simulink model "Sim_OSQP_PC"  (R2025b)
settings: Solver=ode45  StartTime=0.0  StopTime=0.7  FixedStep=Ts/2  RelTol=1e-3
values from neighbouring files (symbols this model uses):
  Ad = evalin('base','Ad')    [PC_OSQP.m]    (also in PC_OSQP_WHAT.m)
  Bd = evalin('base','Bd')    [PC_OSQP.m]    (also in PC_OSQP_WHAT.m)
  Cf = Cf_values(k)    [Init_OSQP_PC.m]    (also in PC_PIControl.m = 1.2e-05)
  Lf = Lf_values(k)    [Init_OSQP_PC.m]    (also in PC_PIControl.m = 0.005)
  Lg = Lg_values(k)    [Init_OSQP_PC.m]    (also in PC_PIControl.m = 0.0033)
  Rf = 0.035    [Init_OSQP_PC.m]    (also in PC_PIControl.m)
  Rg = Rg_values(k)    [Init_OSQP_PC.m]    (also in PC_PIControl.m = 0.84)
  Ts = 1/fs    (= 0.0002)    [Init_OSQP_PC.m]    (also in PC_PIControl.m)
  Vb = Vdc*(sqrt(3)/3)/1.15    [Init_OSQP_PC.m]    (also in PC_PIControl.m)
  Vdc = 300    [Init_OSQP_PC.m]    (also in PC_PIControl.m)
  wb = 2*pi*f    (= 314.159265359)    [Init_OSQP_PC.m]    (also in PC_PIControl.m)
undefined symbols (not defined in the file or in its folder): Bpd, Cd, plecs
libraries: dspsigops x2
settings Model: Creator=ASUS-PC  LastModifiedBy=dfigueroa
settings SolverCC: AllowMultiTaskInputOutput=on  PositivePriorityOrder=on
settings DebuggingCC: IntegerOverflowMsg=error  ParameterPrecisionLossMsg=error  UnderSpecifiedDimensionMsg=warning
settings RTWCC: GPUComputeCapability=3.5

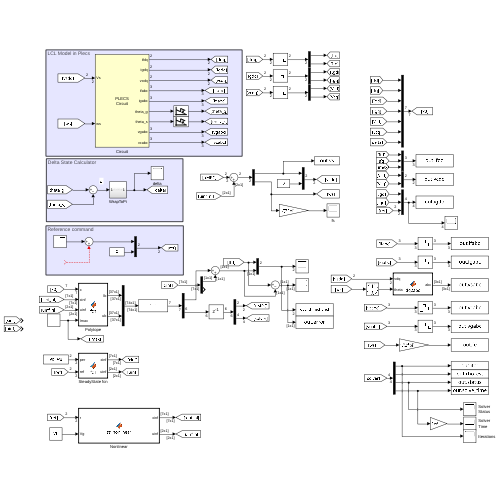
[thumbnail: Simulink's stored preview of the top-level diagram]
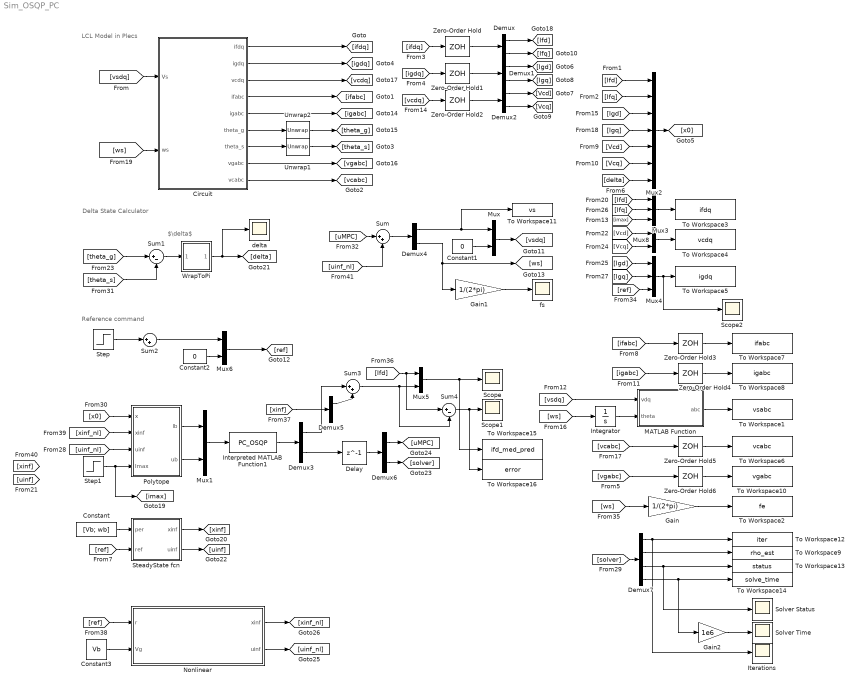
== system Sim_OSQP_PC ==
  note: LCL Model in Plecs
  note: Reference command
  note: $\delta$
  note: Delta State Calculator
  Circuit : Subsystem  LoadFcn=plecs('sl', 200);  InitFcn=plecs('sl', 214);  StartFcn=plecs('sl', 208);  StopFcn=plecs('sl', 209);  mask(PlecsCircuit){PLECSData=<binary blob, 7204 chars, not shown>}
      mask prompts: PLECSData "PLECS Data (Do not delete or modify!)"
      mask init:
      | % PLACE CUSTOM INITIALIZATIONS ABOVE
      | % DO NOT REMOVE
      | plecs('sl', 215);
      | % DO NOT REMOVE
      settings: CopyFcn=plecs('sl', 203);  DeleteFcn=plecs('sl', 205);  UndoDeleteFcn=plecs('sl', 206);  PreSaveFcn=plecs('sl', 211);  PostSaveFcn=plecs('sl', 201);  NameChangeFcn=plecs('sl', 210);  DestroyFcn=plecs('sl', 207);  PreCopyFcn=plecs('sl', 216);  OpenFcn=plecs('sl', 202);  ErrorFcn=plerrorfcn
      mask Help: eval('plecs(''help'', ''qthelp:///creatingacircuit.html'')')
      mask Display: disp('PLECS\nCircuit')
  Constant : Constant  Value=[Vb; wb]  SampleTime=Ts
  Constant1 : Constant  Value=0  SampleTime=Ts
  Constant2 : Constant  Value=0  SampleTime=Ts
  Constant3 : Constant  Value=Vb
  Delay : Delay  DelayLength=1  InitialCondition=0  SampleTime=Ts
  Demux{,1..2,4} (4 alike) : Demux  Outputs=2
  Demux3 : Demux  Outputs=[1;6]
  Demux5 : Demux  Outputs=[1;6]
  Demux6 : Demux  Outputs=[2;4]
  Demux7 : Demux
  Gain : Gain  Gain=1/(2*pi)
  Gain1 : Gain  Gain=1/(2*pi)
  Gain2 : Gain  Gain=1e6
  Integrator : Integrator  WrapState=on
  Interpreted MATLAB Function1 : MATLABFcn  StartFcn=clear PC_OSQP  MATLABFcn=PC_OSQP  OutputDimensions=7
  Iterations : Scope
      settings: Title=Iterations  ActiveDisplayYMinimum=-3.75  ActiveDisplayYMaximum=33.75  YLabel=Iterations Number [-]
  MATLAB Function : MATLAB Function  TreatAsAtomicUnit=on
  Mux{,1,5..6,8} (5 alike) : Mux  Inputs=2
  Mux2 : Mux  Inputs=7
  Mux3 : Mux  Inputs=3
  Mux4 : Mux  Inputs=3
  Nonlinear : MATLAB Function  TreatAsAtomicUnit=on
  Polytope : MATLAB Function  TreatAsAtomicUnit=on
  Scope : Scope
      settings: ActiveDisplayYMinimum=-4.5545615046409651  ActiveDisplayYMaximum=8.000947565725788
  Scope1 : Scope
      settings: ActiveDisplayYMinimum=-0.52018876993310137  ActiveDisplayYMaximum=1.1247691139620895  DataLoggingVariableName=ScopeData6
  Scope2 : Scope
      settings: ActiveDisplayYMinimum=2.349689265196981  ActiveDisplayYMaximum=6.2165319723258836  DataLoggingVariableName=ScopeData7
  Solver Status : Scope
      settings: ActiveDisplayYMinimum=-2.5  ActiveDisplayYMaximum=2.5  DataLoggingVariableName=ScopeData2
  Solver Time : Scope
      settings: Title=Solver Timer  ActiveDisplayYMinimum=-35.6125  ActiveDisplayYMaximum=320.5125  YLabel=Solver Time [\mu s]  DataLoggingVariableName=ScopeData3
  SteadyState fcn : MATLAB Function  TreatAsAtomicUnit=on
  Step : Step  Time=0.2  Before=3  After=5.5  SampleTime=Ts
  Step1 : Step  Time=0.4  Before=7  After=4  SampleTime=Ts
  Sum : Sum  Inputs=|++
  Sum1 : Sum  Inputs=|+-
  Sum2 : Sum  Inputs=|++
  Sum3 : Sum  Inputs=|++
  Sum4 : Sum  Inputs=|+-
  To Workspace1 : ToWorkspace  VariableName=vsabc  SaveFormat=Structure With Time  SampleTime=Ts
  To Workspace10 : ToWorkspace  VariableName=vgabc  SaveFormat=Structure With Time  SampleTime=Ts
  To Workspace11 : ToWorkspace  VariableName=vs  SaveFormat=Structure With Time  SampleTime=Ts
  To Workspace12 : ToWorkspace  VariableName=iter  SaveFormat=Structure With Time  SampleTime=Ts
  To Workspace13 : ToWorkspace  VariableName=status  SaveFormat=Structure With Time  SampleTime=Ts
  To Workspace14 : ToWorkspace  VariableName=solve_time  SaveFormat=Structure With Time  SampleTime=Ts
  To Workspace15 : ToWorkspace  VariableName=ifd_med_pred  SaveFormat=Structure With Time  SampleTime=Ts
  To Workspace16 : ToWorkspace  VariableName=error  SaveFormat=Structure With Time  SampleTime=Ts
  To Workspace2 : ToWorkspace  VariableName=fe  SaveFormat=Structure With Time  SampleTime=Ts
  To Workspace3 : ToWorkspace  VariableName=ifdq  SaveFormat=Structure With Time  SampleTime=Ts
  To Workspace4 : ToWorkspace  VariableName=vcdq  SaveFormat=Structure With Time  SampleTime=Ts
  To Workspace5 : ToWorkspace  VariableName=igdq  SaveFormat=Structure With Time  SampleTime=Ts
  To Workspace6 : ToWorkspace  VariableName=vcabc  SaveFormat=Structure With Time  SampleTime=Ts
  To Workspace7 : ToWorkspace  VariableName=ifabc  SaveFormat=Structure With Time  SampleTime=Ts
  To Workspace8 : ToWorkspace  VariableName=igabc  SaveFormat=Structure With Time  SampleTime=Ts
  To Workspace9 : ToWorkspace  VariableName=rho_est  SaveFormat=Structure With Time  SampleTime=Ts
  Unwrap1 : dspsigops/Unwrap  tol=pi  InputProcessing=Columns as channels (frame based)  running=off
  Unwrap2 : dspsigops/Unwrap  tol=pi  InputProcessing=Columns as channels (frame based)  running=off
  WrapToPi : Subsystem
  Zero-Order Hold{,1..6} (7 alike) : ZeroOrderHold  SampleTime=Ts
  delta : Scope
      settings: ActiveDisplayYMinimum=-1.786361940760036  ActiveDisplayYMaximum=0.36929419889135839  DataLoggingVariableName=ScopeData4
  fs : Scope
      settings: ActiveDisplayYMinimum=43.68062  ActiveDisplayYMaximum=55.78728  DataLoggingVariableName=ScopeData5
  wires:
  [Ifd] -> Mux2/1
  Circuit/8(vgabc) -> [vgabc]
  Circuit/2(igdq) -> [igdq]
  [vsdq] -> Circuit/1(Vs)
  [Vcd] -> Mux2/5
  Circuit/1(ifdq) -> [ifdq]
  Unwrap2/1 -> [theta_g]
  Circuit/5(igabc) -> [igabc]
  Circuit/3(vcdq) -> [vcdq]
  Mux2/1 -> [x0]
  [Ifq] -> Mux2/2
  [ws] -> Circuit/2(ws)
  [Vcq] -> Mux2/6
  [delta] -> Mux2/7
  Unwrap1/1 -> [theta_s]
  Circuit/4(ifabc) -> [ifabc]
  [Igq] -> Mux2/4
  [Igd] -> Mux2/3
  Constant/1 -> SteadyState fcn/1(per)
  [ref] -> SteadyState fcn/2(ref)
  [x0] -> Polytope/1(x)
  Polytope/1(lb) -> Mux1/1
  Polytope/2(ub) -> Mux1/2
  Mux1/1 -> Interpreted MATLAB Function1/1
  Circuit/9(vcabc) -> [vcabc]
  Circuit/6(theta_g) -> Unwrap2/1
  Circuit/7(theta_s) -> Unwrap1/1
  Step1/1 -> [imax], Polytope/4(Imax)
  [theta_s] -> Sum1/2
  Demux7/3 -> Solver Status/1, To Workspace13/1
  Gain2/1 -> Solver Time/1
  Sum/1 -> Demux4/1
  Constant1/1 -> Mux/2
  Gain1/1 -> fs/1
  Sum1/1 -> WrapToPi/1(In1)
  Demux7/4 -> Gain2/1, To Workspace14/1
  Demux4/2 -> Gain1/1, [ws]
  Constant2/1 -> Mux6/2
  Demux7/2 -> To Workspace9/1
  Mux/1 -> [vsdq]
  [theta_g] -> Sum1/1
  Demux7/1 -> Iterations/1, To Workspace12/1
  Mux6/1 -> [ref]
  WrapToPi/1(Out1) -> [delta], delta/1
  Delay/1 -> Demux6/1
  Demux4/1 -> To Workspace11/1, Mux/1
  Zero-Order Hold2/1 -> Demux2/1
  Demux1/2 -> [Igq]
  [vcdq] -> Zero-Order Hold2/1
  Zero-Order Hold1/1 -> Demux1/1
  Demux/1 -> [Ifd]
  Demux2/2 -> [Vcq]
  [ifdq] -> Zero-Order Hold/1
  Demux1/1 -> [Igd]
  Zero-Order Hold/1 -> Demux/1
  Demux2/1 -> [Vcd]
  [igdq] -> Zero-Order Hold1/1
  Demux/2 -> [Ifq]
  [Igq] -> Mux4/2
  [Vcd] -> Mux8/1
  Zero-Order Hold4/1 -> To Workspace8/1
  Gain/1 -> To Workspace2/1
  Zero-Order Hold3/1 -> To Workspace7/1
  Integrator/1 -> MATLAB Function/2(theta)
  [Vcq] -> Mux8/2
  Mux4/1 -> Scope2/1, To Workspace5/1
  [ifabc] -> Zero-Order Hold3/1
  [igabc] -> Zero-Order Hold4/1
  [Ifd] -> Mux3/1
  [ref] -> Mux4/3
  [vgabc] -> Zero-Order Hold6/1
  [Igd] -> Mux4/1
  MATLAB Function/1(abc) -> To Workspace1/1
  [vcabc] -> Zero-Order Hold5/1
  [Ifq] -> Mux3/2
  Zero-Order Hold6/1 -> To Workspace10/1
  [imax] -> Mux3/3
  Zero-Order Hold5/1 -> To Workspace6/1
  Mux3/1 -> To Workspace3/1
  Mux8/1 -> To Workspace4/1
  [ws] -> Integrator/1
  Step/1 -> Sum2/1
  Sum2/1 -> Mux6/1
  ? -> Sum2/2
  [vsdq] -> MATLAB Function/1(vdq)
  SteadyState fcn/1(xinf) -> [xinf]
  SteadyState fcn/2(uinf) -> [uinf]
  [xinf_nl] -> Polytope/2(xinf)
  [uinf_nl] -> Polytope/3(uinf)
  Demux6/2 -> [solver]
  [solver] -> Demux7/1
  Demux6/1 -> [uMPC]
  [uMPC] -> Sum/1
  [uinf_nl] -> Sum/2
  [ws] -> Gain/1
  Interpreted MATLAB Function1/1 -> Demux3/1
  Demux3/2 -> Delay/1
  Demux3/1 -> Sum3/1
  Mux5/1 -> To Workspace15/1, Scope/1
  Sum3/1 -> Sum4/2, Mux5/2
  [xinf] -> Demux5/1
  Demux5/1 -> Sum3/2
  Sum4/1 -> To Workspace16/1, Scope1/1
  [Ifd] -> Sum4/1, Mux5/1
  [ref] -> Nonlinear/1(r)
  Constant3/1 -> Nonlinear/2(Vg)
  Nonlinear/2(uinf) -> [uinf_nl]
  Nonlinear/1(xinf) -> [xinf_nl]

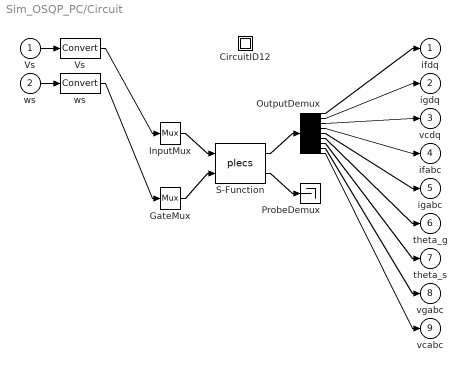
== system Sim_OSQP_PC/Circuit ==
  Vs : Inport  PortDimensions=2
  ws : Inport  Port=2  PortDimensions=1
  " CircuitID12 " : Subsystem
  " GateMux " : Mux  Inputs=[ 1 ]
  " InputMux " : Mux  Inputs=[ 2 ]
  " OutputDemux " : Demux  Outputs=[ 2 2 2 3 3 1 1 3 3 ]
  " ProbeDemux " : Terminator
  " S-Function " : S-Function  FunctionName=plecs  SFunctionDeploymentMode=off  EnableBusSupport=off
  " Vs " : DataTypeConversion
  " ws " : DataTypeConversion
  ifdq : Outport  PortDimensions=2
  igdq : Outport  Port=2  PortDimensions=2
  vcdq : Outport  Port=3  PortDimensions=2
  ifabc : Outport  Port=4  PortDimensions=3
  igabc : Outport  Port=5  PortDimensions=3
  theta_g : Outport  Port=6  PortDimensions=1
  theta_s : Outport  Port=7  PortDimensions=1
  vgabc : Outport  Port=8  PortDimensions=3
  vcabc : Outport  Port=9  PortDimensions=3
  wires:
  " InputMux "/1 -> " S-Function "/1
  " GateMux "/1 -> " S-Function "/2
  " S-Function "/1 -> " OutputDemux "/1
  " S-Function "/2 -> " ProbeDemux "/1
  Vs/1 -> " Vs "/1
  " Vs "/1 -> " InputMux "/1
  ws/1 -> " ws "/1
  " ws "/1 -> " GateMux "/1
  " OutputDemux "/1 -> ifdq/1
  " OutputDemux "/2 -> igdq/1
  " OutputDemux "/3 -> vcdq/1
  " OutputDemux "/4 -> ifabc/1
  " OutputDemux "/5 -> igabc/1
  " OutputDemux "/6 -> theta_g/1
  " OutputDemux "/7 -> theta_s/1
  " OutputDemux "/8 -> vgabc/1
  " OutputDemux "/9 -> vcabc/1

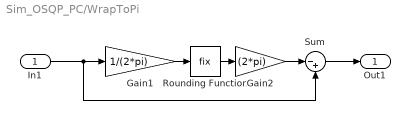
== system Sim_OSQP_PC/WrapToPi ==
  In1 : Inport
  Gain1 : Gain  Gain=1/(2*pi)
  Gain2 : Gain  Gain=(2*pi)
  Rounding Function : Rounding  Operator=fix
  Sum : Sum  Inputs=|-+
  Out1 : Outport
  wires:
  Gain2/1 -> Sum/1
  Gain1/1 -> Rounding Function/1
  Rounding Function/1 -> Gain2/1
  In1/1 -> Sum/2, Gain1/1
  Sum/1 -> Out1/1

== system Sim_OSQP_PC/Circuit/ CircuitID12  ==

== matlab function Sim_OSQP_PC/MATLAB Function ==
  data: vdq input; abc output; theta input
function abc = dq2abc(vdq,theta)
    T = [sin(theta)        -sin(theta)        ;
         cos(theta-2*pi/3) -sin(theta-2*pi/3) ;
         cos(theta+2*pi/3) -sin(theta+2*pi/3)];
    abc = T*vdq;

== matlab function Sim_OSQP_PC/Polytope ==
  data: x input; xinf input; lb output; ub output; uinf input; Imax input; Bd parameter; Vdc parameter
function [lb, ub] = fcn(x, xinf, uinf, Imax, Bd, Vdc)
    [nx,~] = size(Bd); N = 2;

    Mi = [1 0 0 0 0 0 0;
          0 1 0 0 0 0 0];

    a1 = tan(deg2rad(15)); a2 = tan(deg2rad(45)); a3 = tan(deg2rad(75));

    r1 = 1; r2 = 1.366; r3 = 3.7321;
    
    Hi = [a1  1 ;
          a2  1 ;
          a3  1 ;
          a3 -1 ;
          a2 -1 ;
          a1 -1];
 
    xmax = Imax*[r1;
                 r2;
                 r3;
                 r3;
                 r2;
                 r1];
    xmin = -xmax;

    Hv = [1 0 ;
          0 1];
    wmax = 2*pi*70;

    hv = [0.95*(sqrt(3)/3)*Vdc ;
                          wmax];
    
    umax = hv;

    umin = -umax;
    umin(2) = 0 ;

    leq = [-(x - xinf)     ;
            zeros(N*nx, 1)];
    ueq = leq;

    x_uineq = [kron(ones(N,1), xmax - Hi*Mi*xinf)];
    u_uineq = [kron(ones(N,1), umax - Hv*uinf)]   ;
    x_lineq = [kron(ones(N,1), xmin - Hi*Mi*xinf)];
    u_lineq = [kron(ones(N,1), umin - Hv*uinf)]   ;

    lb = [leq     ;
          x_lineq ;
          u_lineq];
    ub = [ueq     ;
          x_uineq ;
          u_uineq];
end

== matlab function Sim_OSQP_PC/SteadyState fcn ==
  data: per input; xinf output; uinf output; ref input; Ad parameter; Cd parameter; Bd parameter; Bpd parameter
function [xinf, uinf] = fcn(per, ref, Ad, Cd, Bd, Bpd)
    H_k = [0 0 1 0 0 0 0;
           0 0 0 1 0 0 0];
    Asolve = [eye(length(Ad)) - Ad   -Bd; 
                    H_k*Cd          zeros(size(Bd,2))];
    Csolve = [ [Bd Bpd]*[0;0;per];
                       ref];
    infty  = linsolve(Asolve,Csolve);
    xinf = infty(1:size(Ad,1));
    uinf = infty(size(Ad,1) + 1:end);
end

== matlab function Sim_OSQP_PC/Nonlinear ==
  data: r input; xinf output; uinf output; Vg input; wb parameter; Lf parameter; Rf parameter; Lg parameter; Rg parameter; Cf parameter
function [xinf, uinf] = ss_nonlinear(r, Vg, wb,Lf,Rf, Lg, Rg, Cf)

rd = r(1); rq = r(2);

z0 = [rd; rq; Vg; 0; 0; Vg];

F = @(z) [
    -Rf*z(1) + wb*Lf*z(2) - z(3) + z(6);                           % ifd eq
    -Rf*z(2) - wb*Lf*z(1) - z(4);                                  % ifq eq
    -Rg*rd   + wb*Lg*rq   - Vg*cos(z(5)) + z(3);                   % vcd from igd
    -Rg*rq   - wb*Lg*rd   - Vg*sin(z(5)) + z(4);                   % vcq from igq
    -rd + z(1) + wb*Cf*z(4);                                       % cap d
    -rq + z(2) - wb*Cf*z(3)                                        % cap q
];

opts = optimoptions('fsolve','Algorithm','levenberg-marquardt');

[zsol,~,~] = fsolve(F, z0, opts);

% pack outputs
ifd   = zsol(1);  ifq = zsol(2);
vcd   = zsol(3);  vcq = zsol(4);
delta = zsol(5);  vsd = zsol(6);

xinf = [ifd; ifq; rd; rq; vcd; vcq; wrapToPi(delta)];
uinf = [vsd; wb];
end
